simulink subsystem "GUIDANCE"  (R2025b)
settings: Solver=VariableStepAuto  StartTime=0.0  StopTime=10.0  RelTol=1e-3
model mask{targetID=0}
  mask prompts: targetID "Target identifier"
libraries: simulink x6, matrix_library x2, vrlib x2
settings Model: Creator=antoniohernandez-rodiciomateos  LastModifiedBy=antoniohernandez-rodiciomateos

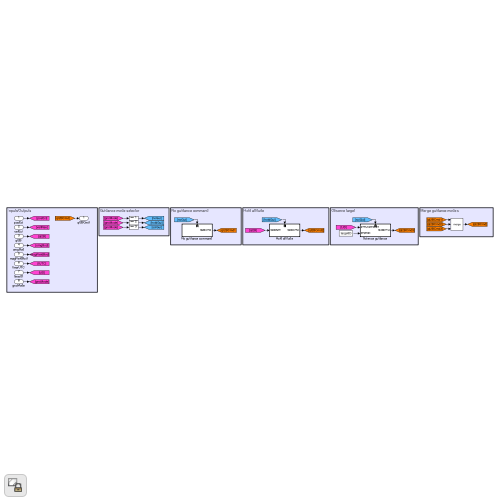
[thumbnail: Simulink's stored preview of the top-level diagram]
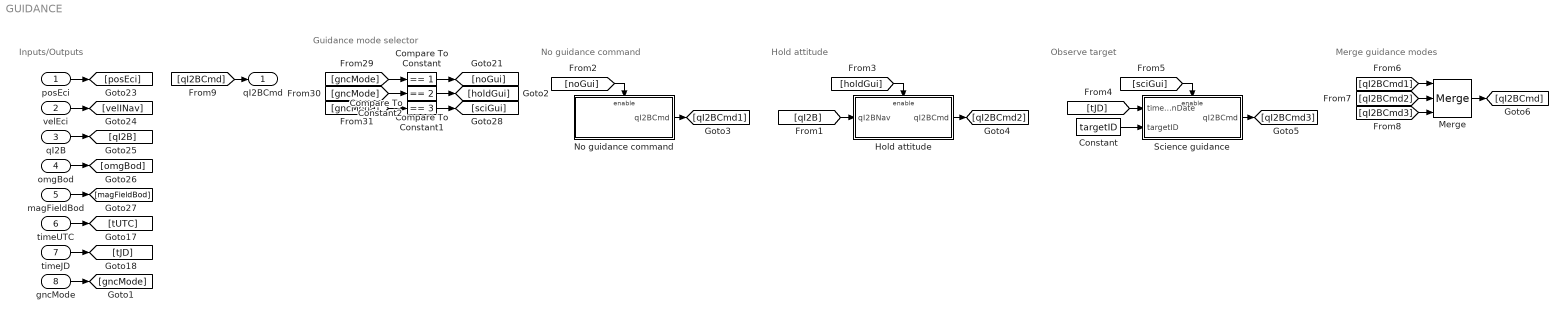
== system GUIDANCE ==
  note: Inputs/Outputs
  note: Guidance mode selector
  note: No guidance command
  note: Hold attitude
  note: Observe target
  note: Merge guidance modes
  posEci : Inport  OutDataTypeStr=double  PortDimensions=[3 1]
  velEci : Inport  Port=2  OutDataTypeStr=double  PortDimensions=[3 1]
  qI2B : Inport  Port=3  OutDataTypeStr=double  PortDimensions=[4 1]
  omgBod : Inport  Port=4  OutDataTypeStr=double  PortDimensions=[3 1]
  magFieldBod : Inport  Port=5  OutDataTypeStr=double  PortDimensions=[3 1]
  timeUTC : Inport  Port=6  OutDataTypeStr=double  PortDimensions=[1 1]
  timeJD : Inport  Port=7  OutDataTypeStr=double  PortDimensions=[1 1]
  gncMode : Inport  Port=8  OutDataTypeStr=double  PortDimensions=[1 1]
  Compare To Constant : simulink/Logic and Bit Operations/Compare To Constant  relop===  const=1  OutDataTypeStr=boolean
  Compare To Constant1 : simulink/Logic and Bit Operations/Compare To Constant  relop===  const=2  OutDataTypeStr=boolean
  Compare To Constant2 : simulink/Logic and Bit Operations/Compare To Constant  relop===  const=3  OutDataTypeStr=boolean
  Constant : Constant  Value=targetID
  Hold attitude : Subsystem
  Merge : Merge  Inputs=3
  No guidance command : Subsystem
  Science guidance : Subsystem
  qI2BCmd : Outport  OutDataTypeStr=double  PortDimensions=[4 1]
  wires:
  posEci/1 -> [posEci]
  velEci/1 -> [velINav]
  qI2B/1 -> [qI2B]
  omgBod/1 -> [omgBod]
  magFieldBod/1 -> [magFieldBod]
  timeUTC/1 -> [tUTC]
  timeJD/1 -> [tJD]
  gncMode/1 -> [gncMode]
  Compare To Constant/1 -> [noGui]
  [gncMode] -> Compare To Constant1/1
  [gncMode] -> Compare To Constant2/1
  Compare To Constant1/1 -> [holdGui]
  [gncMode] -> Compare To Constant/1
  Compare To Constant2/1 -> [sciGui]
  [noGui] -> No guidance command/Enable
  No guidance command/1(qI2BCmd) -> [qI2BCmd1]
  [holdGui] -> Hold attitude/Enable
  Hold attitude/1(qI2BCmd) -> [qI2BCmd2]
  [qI2B] -> Hold attitude/1(qI2BNav)
  [tJD] -> Science guidance/1(timeJulianDate)
  Constant/1 -> Science guidance/2(targetID)
  [sciGui] -> Science guidance/Enable
  Science guidance/1(qI2BCmd) -> [qI2BCmd3]
  Merge/1 -> [qI2BCmd]
  [qI2BCmd1] -> Merge/1
  [qI2BCmd2] -> Merge/2
  [qI2BCmd3] -> Merge/3
  [qI2BCmd] -> qI2BCmd/1

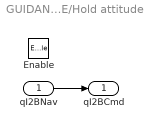
== system GUIDANCE/Hold attitude ==
  qI2BNav : Inport
  Enable : EnablePort
  qI2BCmd : Outport
  wires:
  qI2BNav/1 -> qI2BCmd/1

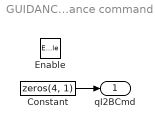
== system GUIDANCE/No guidance command ==
  Enable : EnablePort
  Constant : Constant  Value=zeros(4, 1)
  qI2BCmd : Outport
  wires:
  Constant/1 -> qI2BCmd/1

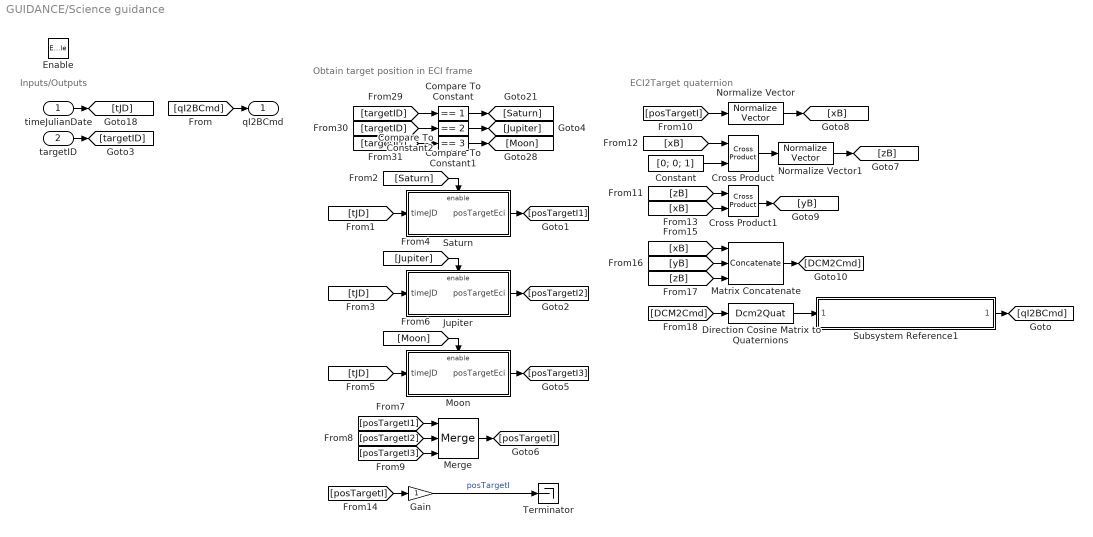
== system GUIDANCE/Science guidance ==
  note: Inputs/Outputs
  note: Obtain target position in ECI frame
  note: ECI2Target quaternion
  timeJulianDate : Inport  OutDataTypeStr=double  PortDimensions=[1 1]
  targetID : Inport  Port=2  OutDataTypeStr=double  PortDimensions=[1 1]
  Enable : EnablePort
  Compare To Constant : simulink/Logic and Bit Operations/Compare To Constant  relop===  const=1  OutDataTypeStr=boolean
  Compare To Constant1 : simulink/Logic and Bit Operations/Compare To Constant  relop===  const=2  OutDataTypeStr=boolean
  Compare To Constant2 : simulink/Logic and Bit Operations/Compare To Constant  relop===  const=3  OutDataTypeStr=boolean
  Constant : Constant  Value=[0; 0; 1]
  Cross Product : matrix_library/Cross Product
  Cross Product1 : matrix_library/Cross Product
  Direction Cosine Matrix to Quaternions : Dcm2Quat
  Gain : Gain
  Jupiter : Subsystem
  Matrix Concatenate : Concatenate  NumInputs=3  Mode=Multidimensional array  ConcatenateDimension=2
  Merge : Merge  Inputs=3
  Moon : Subsystem
  Normalize Vector : vrlib/Utilities/Normalize Vector  maxzero=0
  Normalize Vector1 : vrlib/Utilities/Normalize Vector  maxzero=0
  Saturn : Subsystem
  Subsystem Reference1 : Subsystem  ReferencedSubsystem=quatConventionConverter  conversion=q0 to q4
  Terminator : Terminator
  qI2BCmd : Outport
  wires:
  Gain/1 -> Terminator/1  "posTargetI"
  [posTargetI] -> Gain/1
  Merge/1 -> [posTargetI]
  [posTargetI3] -> Merge/3
  [posTargetI2] -> Merge/2
  [posTargetI1] -> Merge/1
  [Moon] -> Moon/Enable
  Moon/1(posTargetEci) -> [posTargetI3]
  [tJD] -> Moon/1(timeJD)
  [Jupiter] -> Jupiter/Enable
  Jupiter/1(posTargetEci) -> [posTargetI2]
  [tJD] -> Jupiter/1(timeJD)
  Saturn/1(posTargetEci) -> [posTargetI1]
  [tJD] -> Saturn/1(timeJD)
  [Saturn] -> Saturn/Enable
  [targetID] -> Compare To Constant/1
  [targetID] -> Compare To Constant1/1
  Compare To Constant/1 -> [Saturn]
  Compare To Constant2/1 -> [Moon]
  Compare To Constant1/1 -> [Jupiter]
  [targetID] -> Compare To Constant2/1
  targetID/1 -> [targetID]
  timeJulianDate/1 -> [tJD]
  [qI2BCmd] -> qI2BCmd/1
  Cross Product/1 -> Normalize Vector1/1
  Constant/1 -> Cross Product/2
  Cross Product1/1 -> [yB]
  [xB] -> Cross Product1/2
  [posTargetI] -> Normalize Vector/1
  [DCM2Cmd] -> Direction Cosine Matrix to Quaternions/1
  Subsystem Reference1/1 -> [qI2BCmd]
  Normalize Vector1/1 -> [zB]
  Direction Cosine Matrix to Quaternions/1 -> Subsystem Reference1/1
  Normalize Vector/1 -> [xB]
  [xB] -> Cross Product/1
  [zB] -> Cross Product1/1
  [yB] -> Matrix Concatenate/2
  [zB] -> Matrix Concatenate/3
  Matrix Concatenate/1 -> [DCM2Cmd]
  [xB] -> Matrix Concatenate/1

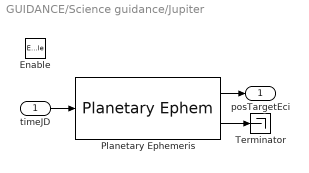
== system GUIDANCE/Science guidance/Jupiter ==
  timeJD : Inport  OutDataTypeStr=double  PortDimensions=[1 1]
  Enable : EnablePort
  Planetary Ephemeris : PlanetaryEphem  target=Jupiter
  Terminator : Terminator
  posTargetEci : Outport  OutDataTypeStr=double  PortDimensions=[3 1]
  wires:
  Planetary Ephemeris/2 -> Terminator/1
  Planetary Ephemeris/1 -> posTargetEci/1
  timeJD/1 -> Planetary Ephemeris/1

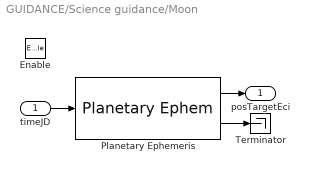
== system GUIDANCE/Science guidance/Moon ==
  timeJD : Inport  OutDataTypeStr=double  PortDimensions=[1 1]
  Enable : EnablePort
  Planetary Ephemeris : PlanetaryEphem
  Terminator : Terminator
  posTargetEci : Outport  OutDataTypeStr=double  PortDimensions=[3 1]
  wires:
  Planetary Ephemeris/2 -> Terminator/1
  Planetary Ephemeris/1 -> posTargetEci/1
  timeJD/1 -> Planetary Ephemeris/1

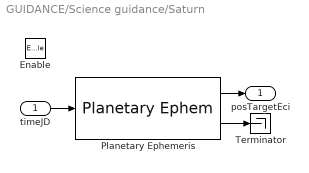
== system GUIDANCE/Science guidance/Saturn ==
  timeJD : Inport  OutDataTypeStr=double  PortDimensions=[1 1]
  Enable : EnablePort
  Planetary Ephemeris : PlanetaryEphem  target=Saturn
  Terminator : Terminator
  posTargetEci : Outport  OutDataTypeStr=double  PortDimensions=[3 1]
  wires:
  Planetary Ephemeris/2 -> Terminator/1
  Planetary Ephemeris/1 -> posTargetEci/1
  timeJD/1 -> Planetary Ephemeris/1
